simulink model "Simulate_NNs"  (Simulink 10.2)
settings: Solver=ode15s  StartTime=0.0  StopTime=30  RelTol=1e-3  EnableMultiTasking=on
libraries: fuzblock x4
settings Model: Creator=Administrator  LastModifiedBy=hunter
settings SolverCC: ZeroCrossControl=DisableAll
settings DataIOCC: LimitDataPoints=on
settings OptimizationCC: ExpressionDepthLimit=2147483647
settings DebuggingCC: SolverPrmCheckMsg=warning  StateNameClashWarn=warning

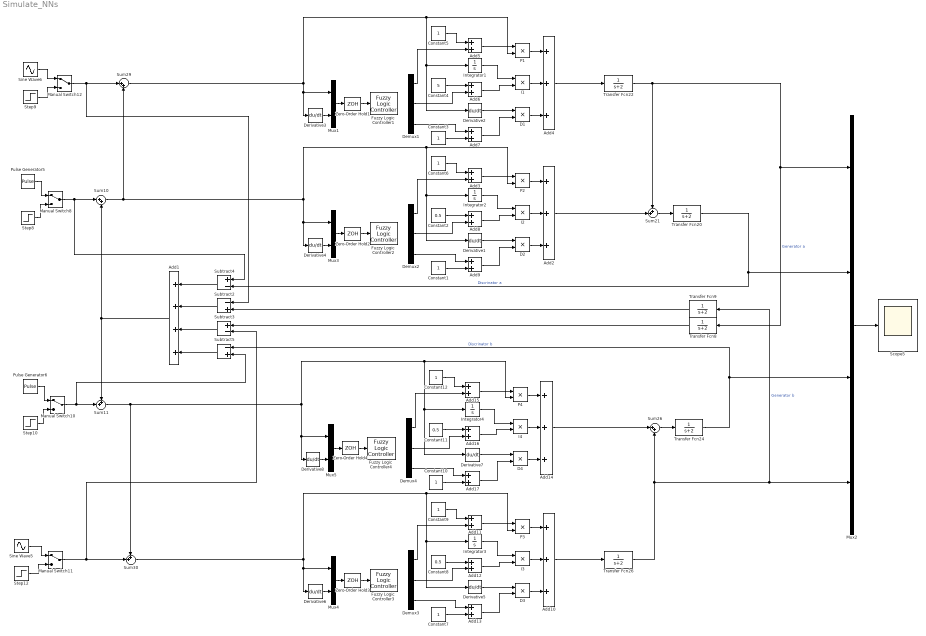
== system Simulate_NNs ==
  Add1 : Sum  Inputs=++++
  Add{2,4,10,14} (4 alike) : Sum  Inputs=+++
  Add{3,5..9,11..13,15..17} (12 alike) : Sum
  Constant{1,3,5..7,9..10,12} (8 alike) : Constant
  Constant11 : Constant  Value=0.5
  Constant2 : Constant  Value=0.5
  Constant4 : Constant  Value=5
  Constant8 : Constant  Value=0.5
  D{1..4} (4 alike) : Product
  Demux{1..4} (4 alike) : Demux  Outputs=3
  Derivative{1..8} (8 alike) : Derivative
  Fuzzy Logic  Controller{1..4} (4 alike) : fuzblock/Fuzzy Logic  Controller  FIS="\"fuzzypidCycleGAN\""  OutputSampleNumber=101  DataType=double  FuzzifiedInputs=off  RuleFiringStrengths=off  RuleOutputs=off  AggregatedOutputs=off  SimulateUsing=Interpreted execution  OutOfRangeInputValueMessage=warning  NoRuleFiredMessage=warning  EmptyOutputFuzzySetMessage=warning
  I{1..4} (4 alike) : Product
  Integrator{1..4} (4 alike) : Integrator
  Manual Switch{8,10..12} (4 alike) : ManualSwitch
  Mux{1,3..5} (4 alike) : Mux  Inputs=2
  Mux2 : Mux
  P{1..4} (4 alike) : Product
  Pulse Generator5 : DiscretePulseGenerator  PulseType=Time based  Period=10  PulseWidth=50
  Pulse Generator6 : DiscretePulseGenerator  PulseType=Time based  Period=10  PulseWidth=50
  Scope5 : Scope
  Sine Wave5 : Sin  Frequency=pi*0.2  Phase=pi  SampleTime=0
  Sine Wave6 : Sin  Frequency=pi*0.2  SampleTime=0
  Step10 : Step  Time=0  SampleTime=0
  Step12 : Step  Time=0  SampleTime=0
  Step8 : Step  Time=0  SampleTime=0
  Step9 : Step  Time=0  After=-1  SampleTime=0
  Subtract2 : Sum  Inputs=-+
  Subtract3 : Sum  Inputs=+-
  Subtract4 : Sum  Inputs=+-
  Subtract5 : Sum  Inputs=-+
  Sum10 : Sum  Inputs=|++
  Sum11 : Sum  Inputs=++|
  Sum21 : Sum  Inputs=++|
  Sum26 : Sum  Inputs=|++
  Sum29 : Sum  Inputs=|++
  Sum30 : Sum  Inputs=++|
  Transfer Fcn{8..9,20,22,24,26} (6 alike) : TransferFcn  Denominator=[1 2]
  Zero-Order Hold{1..4} (4 alike) : ZeroOrderHold
  wires:
  Transfer Fcn26/1 -> Transfer Fcn9/1, Mux2/4, Sum26/2  "Generator b"
  Mux2/1 -> Scope5/1
  Add4/1 -> Transfer Fcn22/1
  Transfer Fcn20/1 -> Subtract4/2, Mux2/2  "Discrinator a"
  Sum26/1 -> Transfer Fcn24/1
  Transfer Fcn9/1 -> Subtract2/2
  Sine Wave5/1 -> Manual Switch11/1
  Manual Switch10/1 -> Subtract5/2, Sum11/2
  Transfer Fcn24/1 -> Subtract5/1, Mux2/3  "Discrinator b"
  Add10/1 -> Transfer Fcn26/1
  Subtract5/1 -> Add1/4
  Add14/1 -> Sum26/1
  Subtract4/1 -> Add1/1
  Manual Switch11/1 -> Subtract3/2, Sum30/2
  Manual Switch12/1 -> Subtract2/1, Sum29/1
  Manual Switch8/1 -> Subtract4/1, Sum10/1
  Transfer Fcn8/1 -> Subtract3/1
  Subtract2/1 -> Add1/2
  Pulse Generator5/1 -> Manual Switch8/1
  Add2/1 -> Sum21/2
  Subtract3/1 -> Add1/3
  Sine Wave6/1 -> Manual Switch12/1
  Sum21/1 -> Transfer Fcn20/1
  Step12/1 -> Manual Switch11/2
  Step10/1 -> Manual Switch10/2
  Pulse Generator6/1 -> Manual Switch10/1
  Add1/1 -> Sum11/1, Sum10/2
  Transfer Fcn22/1 -> Sum21/1, Transfer Fcn8/1, Mux2/1  "Generator a"
  Step9/1 -> Manual Switch12/2
  Step8/1 -> Manual Switch8/2
  Constant4/1 -> Add6/1
  Add6/1 -> I1/2
  Demux1/2 -> Add6/2
  Constant3/1 -> Add7/2
  P1/1 -> Add4/1
  Integrator1/1 -> I1/1
  I1/1 -> Add4/2
  Zero-Order Hold1/1 -> Fuzzy Logic  Controller1/1
  Mux1/1 -> Zero-Order Hold1/1
  D1/1 -> Add4/3
  Demux1/3 -> Add7/1
  Add5/1 -> P1/1
  Derivative2/1 -> D1/1
  Constant5/1 -> Add5/1
  Add7/1 -> D1/2
  Derivative3/1 -> Mux1/2
  Demux1/1 -> Add5/2
  Sum29/1 -> Derivative2/1, Integrator1/1, P1/2, Derivative3/1, Mux1/1
  Constant2/1 -> Add8/1
  Add8/1 -> I2/2
  Demux2/2 -> Add8/2
  Constant1/1 -> Add9/2
  P2/1 -> Add2/1
  Integrator2/1 -> I2/1
  I2/1 -> Add2/2
  Zero-Order Hold2/1 -> Fuzzy Logic  Controller2/1
  Mux3/1 -> Zero-Order Hold2/1
  D2/1 -> Add2/3
  Demux2/3 -> Add9/1
  Add3/1 -> P2/1
  Derivative1/1 -> D2/1
  Constant6/1 -> Add3/1
  Add9/1 -> D2/2
  Derivative4/1 -> Mux3/2
  Demux2/1 -> Add3/2
  Sum10/1 -> Derivative1/1, Integrator2/1, P2/2, Derivative4/1, Mux3/1, Sum29/2
  Constant8/1 -> Add12/1
  Add12/1 -> I3/2
  Demux3/2 -> Add12/2
  Constant7/1 -> Add13/2
  P3/1 -> Add10/1
  Integrator3/1 -> I3/1
  I3/1 -> Add10/2
  Zero-Order Hold3/1 -> Fuzzy Logic  Controller3/1
  Mux4/1 -> Zero-Order Hold3/1
  D3/1 -> Add10/3
  Demux3/3 -> Add13/1
  Add11/1 -> P3/1
  Derivative5/1 -> D3/1
  Constant9/1 -> Add11/1
  Add13/1 -> D3/2
  Derivative6/1 -> Mux4/2
  Demux3/1 -> Add11/2
  Sum30/1 -> Derivative5/1, Integrator3/1, P3/2, Derivative6/1, Mux4/1
  Constant11/1 -> Add16/1
  Add16/1 -> I4/2
  Demux4/2 -> Add16/2
  Constant10/1 -> Add17/2
  P4/1 -> Add14/1
  Integrator4/1 -> I4/1
  I4/1 -> Add14/2
  Zero-Order Hold4/1 -> Fuzzy Logic  Controller4/1
  Mux5/1 -> Zero-Order Hold4/1
  D4/1 -> Add14/3
  Demux4/3 -> Add17/1
  Add15/1 -> P4/1
  Derivative7/1 -> D4/1
  Constant12/1 -> Add15/1
  Add17/1 -> D4/2
  Derivative8/1 -> Mux5/2
  Demux4/1 -> Add15/2
  Sum11/1 -> Derivative7/1, Integrator4/1, P4/2, Derivative8/1, Mux5/1, Sum30/1
